simulink subsystem "supervisor"  (R2024a)
settings: Solver=VariableStepAuto  StartTime=0.0  StopTime=10.0  RelTol=1e-3
settings Model: Creator=User  LastModifiedBy=User

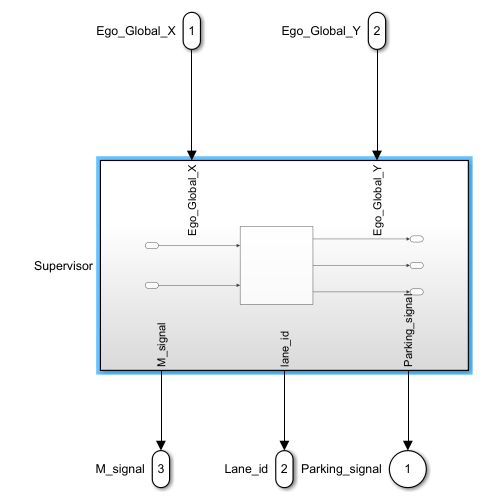
[thumbnail: Simulink's stored preview of the top-level diagram]
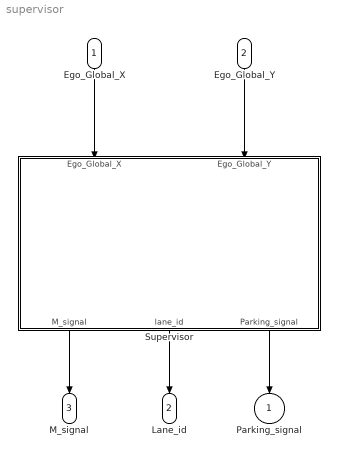
== system supervisor ==
  Ego_Global_X : Inport
  Ego_Global_Y : Inport  Port=2
  Supervisor : Subsystem
  Parking_signal : Outport
  Lane_id : Outport  Port=2
  M_signal : Outport  Port=3
  wires:
  Supervisor/3(Parking_signal) -> Parking_signal/1
  Ego_Global_X/1 -> Supervisor/1(Ego_Global_X)
  Ego_Global_Y/1 -> Supervisor/2(Ego_Global_Y)
  Supervisor/2(lane_id) -> Lane_id/1
  Supervisor/1(M_signal) -> M_signal/1

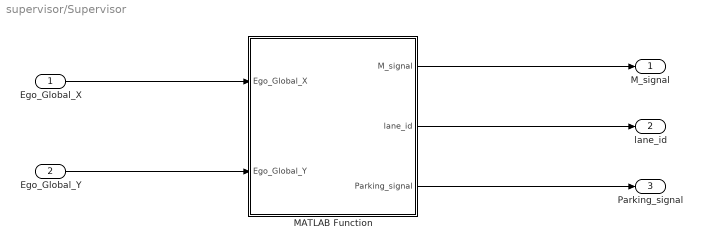
== system supervisor/Supervisor ==
  Ego_Global_X : Inport
  Ego_Global_Y : Inport  Port=2
  MATLAB Function : MATLAB Function  TreatAsAtomicUnit=on
  M_signal : Outport
  lane_id : Outport  Port=2
  Parking_signal : Outport  Port=3
  wires:
  Ego_Global_X/1 -> MATLAB Function/1(Ego_Global_X)
  Ego_Global_Y/1 -> MATLAB Function/2(Ego_Global_Y)
  MATLAB Function/1(M_signal) -> M_signal/1
  MATLAB Function/2(lane_id) -> lane_id/1
  MATLAB Function/3(Parking_signal) -> Parking_signal/1

== matlab function supervisor/Supervisor/MATLAB Function ==
  data: M_signal output; lane_id output; Ego_Global_X input; Parking_signal output; Ego_Global_Y input
function [M_signal, lane_id, Parking_signal]= supervisor(Ego_Global_X, Ego_Global_Y)

[M_signal, lane_id, Parking_signal] = supervisor_fcn(Ego_Global_X, Ego_Global_Y);
end
